simulink model "Prototype_DCS_Simlulink"  (R2018a)
settings: Solver=ode45  StartTime=0.0  StopTime=20  RelTol=1e-3
values from neighbouring files (symbols this model uses):
  A = [A_CAME; A_IKE; A_CLME]    [Prototype.m]    (also in USV1_PID_Fuzzy_Parameters.m = Mass\(-Coriolis - D_l))
  B = [B_CAME; B_IKE; B_CLME]    [Prototype.m]    (also in USV1_PID_Fuzzy_Parameters.m = Mass\F)
  C = eye(9)    [Prototype.m]    (also in USV1_PID_Fuzzy_Parameters.m = eye(4))
  Condition = [0;0;0;0.1;0.1;0;0;0;0]    [Prototype.m]    (also in USV1_PID_Fuzzy_Parameters.m = [1; 0; 0; 3*pi/4])
  D = zeros(9,4)    [Prototype.m]    (also in USV1_PID_Fuzzy_Parameters.m = [ 0  0  0 ;       0  0  0 ;       0  0  0 ;       0  0  0 ])
  g = 9.81    [Prototype.m]
  m = 0.175    [Prototype.m]    (also in USV1_PID_Fuzzy_Parameters.m = 150)
settings Model: Creator=admin  LastModifiedBy=MyPC

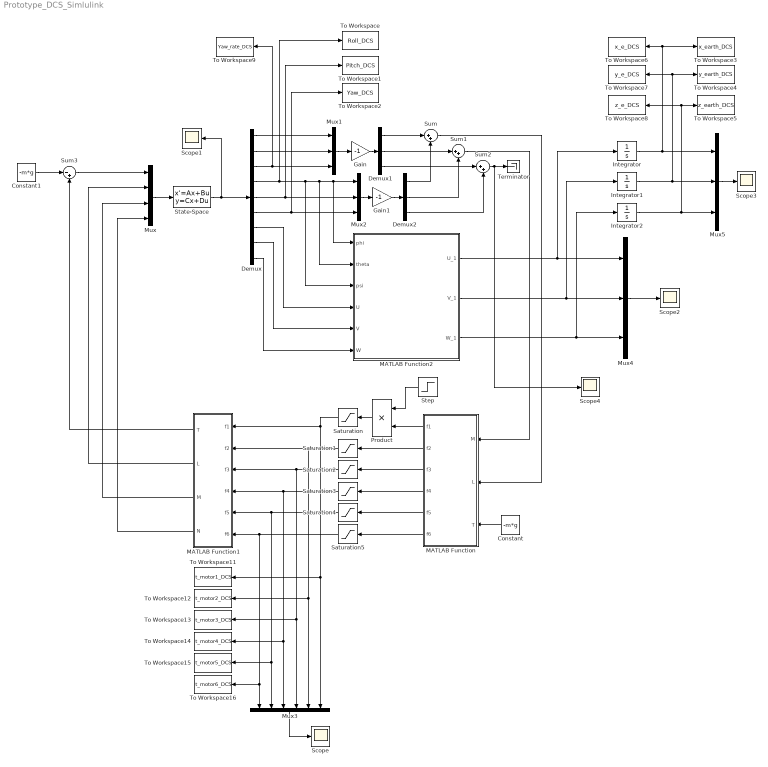
== system Prototype_DCS_Simlulink ==
  Constant : Constant  Value=-m*g
  Constant1 : Constant  Value=-m*g
  Demux : Demux  Outputs=9
  Demux1 : Demux  Outputs=3
  Demux2 : Demux  Outputs=3
  Gain : Gain  Gain=-1
  Gain1 : Gain  Gain=-1
  Integrator : Integrator
  Integrator1 : Integrator
  Integrator2 : Integrator
  MATLAB Function : MATLAB Function  TreatAsAtomicUnit=on
  MATLAB Function1 : MATLAB Function  TreatAsAtomicUnit=on
  MATLAB Function2 : MATLAB Function  TreatAsAtomicUnit=on
  Mux : Mux
  Mux{1..2,4..5} (4 alike) : Mux  Inputs=3
  Mux3 : Mux  Inputs=6
  Product : Product
  Saturation{,1..5} (6 alike) : Saturate  UpperLimit=6  LowerLimit=0
  Scope{,1..4} (5 alike) : Scope
  State-Space : StateSpace  A=A  B=B  C=C  D=D  InitialCondition=Condition
  Step : Step  Before=1  After=0  SampleTime=0
  Sum : Sum  Inputs=|++
  Sum1 : Sum  Inputs=|++
  Sum2 : Sum  Inputs=|++
  Sum3 : Sum  Inputs=|-+
  Terminator : Terminator
  To Workspace : ToWorkspace  VariableName=Roll_DCS  SaveFormat=Timeseries  SampleTime=-1
  To Workspace1 : ToWorkspace  VariableName=Pitch_DCS  SaveFormat=Timeseries  SampleTime=-1
  To Workspace11 : ToWorkspace  VariableName=t_motor1_DCS  SaveFormat=Timeseries  SampleTime=-1
  To Workspace12 : ToWorkspace  VariableName=t_motor2_DCS  SaveFormat=Timeseries  SampleTime=-1
  To Workspace13 : ToWorkspace  VariableName=t_motor3_DCS  SaveFormat=Timeseries  SampleTime=-1
  To Workspace14 : ToWorkspace  VariableName=t_motor4_DCS  SaveFormat=Timeseries  SampleTime=-1
  To Workspace15 : ToWorkspace  VariableName=t_motor5_DCS  SaveFormat=Timeseries  SampleTime=-1
  To Workspace16 : ToWorkspace  VariableName=t_motor6_DCS  SaveFormat=Timeseries  SampleTime=-1
  To Workspace2 : ToWorkspace  VariableName=Yaw_DCS  SaveFormat=Timeseries  SampleTime=-1
  To Workspace3 : ToWorkspace  VariableName=x_earth_DCS  SaveFormat=Timeseries  SampleTime=-1
  To Workspace4 : ToWorkspace  VariableName=y_earth_DCS  SaveFormat=Timeseries  SampleTime=-1
  To Workspace5 : ToWorkspace  VariableName=z_earth_DCS  SaveFormat=Timeseries  SampleTime=-1
  To Workspace6 : ToWorkspace  VariableName=x_e_DCS  SampleTime=-1
  To Workspace7 : ToWorkspace  VariableName=y_e_DCS  SampleTime=-1
  To Workspace8 : ToWorkspace  VariableName=z_e_DCS  SampleTime=-1
  To Workspace9 : ToWorkspace  VariableName=Yaw_rate_DCS  SaveFormat=Timeseries  SampleTime=-1
  wires:
  State-Space/1 -> Demux/1, Scope1/1
  Mux/1 -> State-Space/1
  Demux/1 -> Mux1/1
  Demux/2 -> Mux1/2
  Demux/3 -> To Workspace9/1, Mux1/3
  Demux/4 -> To Workspace/1, MATLAB Function2/3(psi), MATLAB Function2/2(theta), MATLAB Function2/1(phi), Mux2/1
  Demux/5 -> To Workspace1/1, Mux2/2
  Mux1/1 -> Gain/1
  Mux2/1 -> Gain1/1
  Gain/1 -> Demux1/1
  Gain1/1 -> Demux2/1
  Demux1/1 -> Sum/1
  Demux2/1 -> Sum/2
  Demux1/2 -> Sum1/1
  Demux2/2 -> Sum1/2
  Demux1/3 -> Sum2/1
  Demux2/3 -> Sum2/2
  Constant/1 -> MATLAB Function/3(T)
  MATLAB Function/2(f2) -> Saturation1/1
  MATLAB Function/3(f3) -> Saturation2/1
  MATLAB Function/4(f4) -> Saturation3/1
  MATLAB Function/5(f5) -> Saturation4/1
  MATLAB Function/6(f6) -> Saturation5/1
  Saturation5/1 -> To Workspace16/1, Mux3/1, MATLAB Function1/6(f6)
  Saturation/1 -> To Workspace11/1, Mux3/6, MATLAB Function1/1(f1)
  Saturation1/1 -> To Workspace12/1, Mux3/5, MATLAB Function1/2(f2)
  Saturation2/1 -> To Workspace13/1, Mux3/4, MATLAB Function1/3(f3)
  Saturation3/1 -> To Workspace14/1, Mux3/3, MATLAB Function1/4(f4)
  Saturation4/1 -> To Workspace15/1, Mux3/2, MATLAB Function1/5(f5)
  MATLAB Function1/4(N) -> Mux/4
  MATLAB Function1/3(M) -> Mux/3
  MATLAB Function1/2(L) -> Mux/2
  MATLAB Function1/1(T) -> Sum3/2
  Sum3/1 -> Mux/1
  Constant1/1 -> Sum3/1
  Mux3/1 -> Scope/1
  Product/1 -> Saturation/1
  MATLAB Function/1(f1) -> Product/2
  Step/1 -> Product/1
  Demux/9 -> MATLAB Function2/6(W)
  Demux/8 -> MATLAB Function2/5(V)
  Demux/7 -> MATLAB Function2/4(U)
  MATLAB Function2/1(U_1) -> Mux4/1, Integrator/1
  MATLAB Function2/2(V_1) -> Mux4/2, Integrator1/1
  MATLAB Function2/3(W_1) -> Integrator2/1, Mux4/3
  Mux4/1 -> Scope2/1
  Integrator1/1 -> To Workspace7/1, To Workspace4/1, Mux5/2
  Integrator/1 -> To Workspace6/1, To Workspace3/1, Mux5/1
  Integrator2/1 -> To Workspace8/1, To Workspace5/1, Mux5/3
  Mux5/1 -> Scope3/1
  Sum/1 -> MATLAB Function/2(L)
  Sum1/1 -> MATLAB Function/1(M)
  Demux/6 -> To Workspace2/1, Mux2/3
  Sum2/1 -> Scope4/1, Terminator/1

== matlab function Prototype_DCS_Simlulink/MATLAB Function1 ==
  data: f1 input; T output; f2 input; f3 input; f4 input; f5 input; f6 input; L output; M output; N output
function [T,L,M,N] = fcn(f1,f2,f3,f4,f5,f6)
d = 0.1;
k = 0.1;
H = [ -1 -1 -1 -1 -1 -1 ;...
      0 -d*sqrt(3)/2 -d*sqrt(3)/2 0 d*sqrt(3)/2 d*sqrt(3)/2;...
      d d/2 -d/2 -d -d/2 d/2;...
      -k k -k k -k k];

F = H*[f1;f2;f3;f4;f5;f6];

T = F(1);
L = F(2);
M = F(3);
N = F(4);

== matlab function Prototype_DCS_Simlulink/MATLAB Function ==
  data: M input; L input; f1 output; T input; f2 output; f3 output; f4 output; f5 output; f6 output
function [f1,f2,f3,f4,f5,f6] = fcn(M, L, T)
m = 0.175;
g = 9.81;
d = 0.1;
n1 = 0;
n2 = 1;
n3 = 1;
n4 = 1;
n5 = 1;
n6 = 1;
H_DCS = [ -n1 -n2 -n3 -n4 -n5 -n6 ;...
      0 -n2*d*sqrt(3)/2 -n3*d*sqrt(3)/2 0 n5*d*sqrt(3)/2 n6*d*sqrt(3)/2;...
      n1*d n2*d/2 -n3*d/2 -n4*d -n5*d/2 n6*d/2];

A = (H_DCS.')/(H_DCS*(H_DCS.'));
  
B = [T;L;M];

X = A*B;

f1 = X(1);
f2 = X(2);
f3 = X(3);
f4 = X(4);
f5 = X(5);
f6 = X(6);

== matlab function Prototype_DCS_Simlulink/MATLAB Function2 ==
  data: phi input; U_1 output; theta input; psi input; U input; V input; W input; V_1 output; W_1 output
function [U_1, V_1, W_1] = fcn(phi, theta, psi, U, V, W)

U_1 = U*cos(psi)*cos(theta) +...
      V*( -sin(psi)*cos(phi) + cos(psi)*sin(theta)*sin(phi)) +...
      W*( sin(psi)*sin(phi) + cos(psi)*sin(theta)*cos(phi));

V_1 = U*sin(psi)*cos(theta) +...
      V*( cos(psi)*cos(phi) + sin(psi)*sin(theta)*sin(phi)) +...
      W*( -sin(phi)*cos(psi) + sin(psi)*sin(theta)*cos(phi));

W_1 = U*(-sin(theta))+...
      V*(cos(theta)*sin(phi))+...
      W*(cos(theta)*cos(phi));
